simulink model "ysw3_49"  (R2014a)
settings: Solver=ode45  StartTime=0.0  StopTime=10.0  RelTol=1e-3
settings Model: Creator=Administrator  LastModifiedBy=Administrator

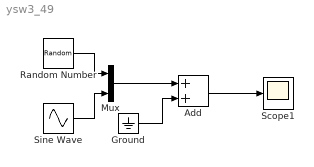
== system ysw3_49 ==
  Add : Sum
  Ground : Ground
  Mux : Mux  Inputs=2
  Random Number : RandomNumber  SampleTime=0.1
  Scope1 : Scope
      settings: TimeRange=10
  Sine Wave : Sin  SampleTime=0.1
  wires:
  Random Number/1 -> Mux/1
  Sine Wave/1 -> Mux/2
  Add/1 -> Scope1/1
  Mux/1 -> Add/1
  Ground/1 -> Add/2
